simulink model "verify_Flow_Mixer_mdl"  (R2016b)
settings: Solver=ode45  StartTime=0.0  StopTime=600  MaxStep=1  RelTol=1e-3  EnableMultiTasking=on
libraries: carnot x8, simulink x2
settings Model: Creator=drhf  LastModifiedBy=drhf
settings DataIOCC: SaveFormat=Array  SignalLoggingSaveFormat=ModelDataLogs
settings OptimizationCC: ExpressionDepthLimit=2147483647  LifeSpan=inf
settings DebuggingCC: UnderspecifiedInitializationDetection=Classic  MergeDetectMultiDrivingBlocksExec=none  SolverPrmCheckMsg=warning  FcnCallInpInsideContextMsg=warning  StateNameClashWarn=warning  SFUnexpectedBacktrackingDiag=warning  SFNoUnconditionalDefaultTransitionDiag=warning  SFExecutionAtInitializationDiag=none
settings HardwareCC: ProdBitPerPointer=32  ProdBitPerSizeT=32  ProdBitPerPtrDiffT=32  ProdLargestAtomicFloat=None  ProdIntDivRoundTo=Undefined  ProdEndianess=Unspecified  ProdWordSize=32  ProdHWDeviceType=32-bit Generic
settings ModelReferenceCC: PropagateSignalLabelsOutOfModel=off
settings GRTTargetCC: TargetLangStandard=C89/C90 (ANSI)  GeneratePreprocessorConditionals=Disable all  CombineOutputUpdateFcns=off  GRTInterface=on
settings ConfigComp: CovMetricSettings=dw  CovHtmlReporting=on  CovSaveCumulativeToWorkspaceVar=on  CovSaveSingleToWorkspaceVar=on  CovExternalEMLEnable=off

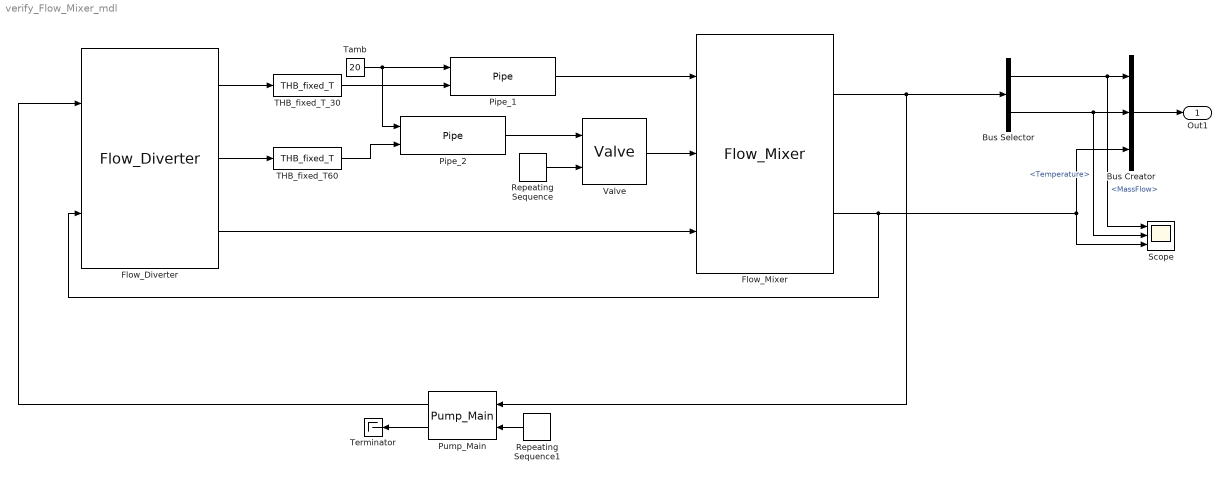
== system verify_Flow_Mixer_mdl ==
  Bus Creator : BusCreator  Inputs=3
  Bus Selector : BusSelector  OutputSignals=MassFlow,Temperature
  Flow_Diverter : carnot/Hydraulics/Flow_Diverter
  Flow_Mixer : carnot/Hydraulics/Flow_Mixer  t=10
  Pipe_1 : carnot/Hydraulics/Pipe  dia=0.02  len=10  hgt=5  uloss=100/20/10  cond=0  cwall=1000  t0=20  lin=100/0.2  qua=100/0.2^2  nodes=10
  Pipe_2 : carnot/Hydraulics/Pipe  dia=0.02  len=10  hgt=5  uloss=100/20/10  cond=0  cwall=1000  t0=20  lin=100/0.2  qua=100/0.2^2  nodes=10
  Pump_Main : carnot/Hydraulics/Pump_Main  a0=2.7e4  a1=-1.2e4  a2=0%-3e-3  dia=0.025  t1=5  p0=3e5  IDchk=off  fluid_id=Water  mix=0  ua=1  mcp=500  tamb=20
  Repeating Sequence : simulink/Sources/Repeating Sequence  rep_seq_t=[0 100 180 200]  rep_seq_y=[1 1 0 0]
  Repeating Sequence1 : simulink/Sources/Repeating Sequence  rep_seq_t=[ 0 300 300+eps(300) 400 400+eps(400) 600]  rep_seq_y=[ 1 1 0+0*eps(300) 0 1+0*eps(400) 1]
  Scope : Scope  NumInputPorts=3
  THB_fixed_T60 : carnot/Source/Simple/THB_fixed_T  t=60
  THB_fixed_T_30 : carnot/Source/Simple/THB_fixed_T  t=30
  Tamb : Constant  Value=20
  Terminator : Terminator
  Valve : carnot/Hydraulics/Valve  pos_values=[0 0.1 1]  dp_values=[1e6 1e6 1]
  Out1 : Outport
  wires:
  Bus Creator/1 -> Out1/1
  Flow_Mixer/1 -> Pump_Main/1, Bus Selector/1
  Bus Selector/1 -> Scope/1, Bus Creator/1  "<MassFlow>"
  Bus Selector/2 -> Scope/2, Bus Creator/2  "<Temperature>"
  Flow_Mixer/2 -> Flow_Diverter/2, Scope/3, Bus Creator/3
  Tamb/1 -> Pipe_1/1, Pipe_2/1
  Pipe_2/1 -> Valve/1
  Repeating Sequence/1 -> Valve/2
  Pipe_1/1 -> Flow_Mixer/1
  THB_fixed_T_30/1 -> Pipe_1/2
  THB_fixed_T60/1 -> Pipe_2/2
  Valve/1 -> Flow_Mixer/2
  Flow_Diverter/1 -> THB_fixed_T_30/1
  Flow_Diverter/2 -> THB_fixed_T60/1
  Flow_Diverter/3 -> Flow_Mixer/3
  Repeating Sequence1/1 -> Pump_Main/2
  Pump_Main/2 -> Terminator/1
  Pump_Main/1 -> Flow_Diverter/1
